simulink model "Button_bouncing"  (R2025b)
settings: Solver=VariableStepAuto  StartTime=0.0  StopTime=100  RelTol=1e-3
libraries: simulink x10, simulink_extras x2
settings Model: Creator=akame  LastModifiedBy=akame

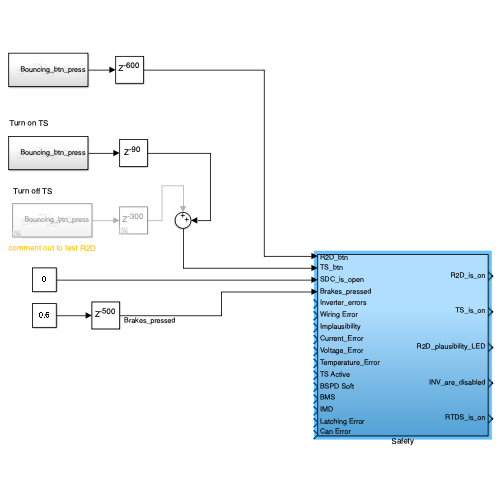
[thumbnail: Simulink's stored preview of the top-level diagram]
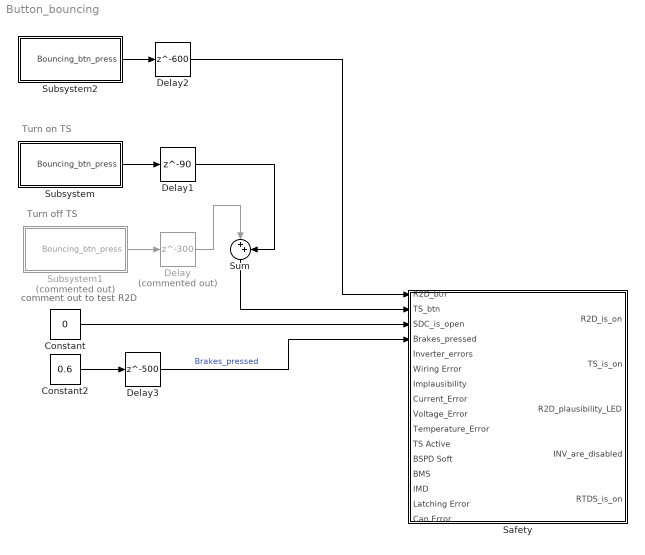
== system Button_bouncing ==
  note: Turn on TS
  note: Turn off TS
  note: comment out to test R2D
  Constant : Constant  Value=0
  Constant2 : Constant  Value=0.6
  Delay : Delay  Commented=on  DelayLength=300
  Delay1 : Delay  DelayLength=90
  Delay2 : Delay  DelayLength=600
  Delay3 : Delay  DelayLength=500
  Safety : Subsystem
  Subsystem : Subsystem
  Subsystem1 : Subsystem  Commented=on
  Subsystem2 : Subsystem
  Sum : Sum  Inputs=|++
  wires:
  Delay1/1 -> Sum/2
  Subsystem1/1(Bouncing_btn_press) -> Delay/1
  Subsystem/1(Bouncing_btn_press) -> Delay1/1
  Delay/1 -> Sum/1
  Sum/1 -> Safety/2(TS_btn)
  Constant/1 -> Safety/3(SDC_is_open)
  Subsystem2/1(Bouncing_btn_press) -> Delay2/1
  Delay2/1 -> Safety/1(R2D_btn)
  Constant2/1 -> Delay3/1
  Delay3/1 -> Safety/4(Brakes_pressed)  "Brakes_pressed"

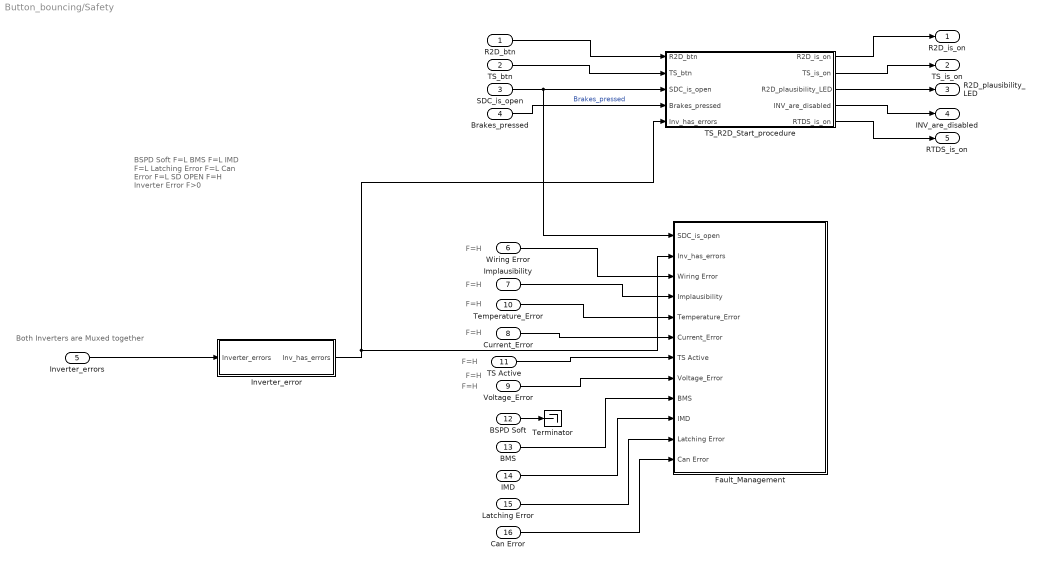
== system Button_bouncing/Safety ==
  note: Both Inverters are Muxed together
  note: F=H
  note: F=H
  note: F=H
  note: F=H
  note: F=H
  note: F=H
  note: F=H
  note: BSPD Soft		F=L
      | BMS			F=L
      | IMD				F=L
      | Latching Error	F=L
      | Can Error		F=L
      | SD OPEN		F=H
      | Inverter Error		F>0
  R2D_btn : Inport
  TS_btn : Inport  Port=2
  SDC_is_open : Inport  Port=3
  Brakes_pressed : Inport  Port=4
  Inverter_errors : Inport  Port=5
  Wiring Error : Inport  Port=6
  Implausibility : Inport  Port=7
  Current_Error : Inport  Port=8
  Voltage_Error : Inport  Port=9
  Temperature_Error : Inport  Port=10
  TS Active : Inport  Port=11
  BSPD Soft : Inport  Port=12
  BMS : Inport  Port=13
  IMD : Inport  Port=14
  Latching Error : Inport  Port=15
  Can Error : Inport  Port=16
  Fault_Management : Subsystem
  Inverter_error : Subsystem
  TS_R2D_Start_procedure : Subsystem
  Terminator : Terminator
  R2D_is_on : Outport
  TS_is_on : Outport  Port=2
  R2D_plausibility_LED : Outport  Port=3
  INV_are_disabled : Outport  Port=4
  RTDS_is_on : Outport  Port=5
  wires:
  TS_btn/1 -> TS_R2D_Start_procedure/2(TS_btn)
  SDC_is_open/1 -> Fault_Management/1(SDC_is_open), TS_R2D_Start_procedure/3(SDC_is_open)
  Brakes_pressed/1 -> TS_R2D_Start_procedure/4(Brakes_pressed)  "Brakes_pressed"
  R2D_btn/1 -> TS_R2D_Start_procedure/1(R2D_btn)
  Inverter_error/1(Inv_has_errors) -> Fault_Management/2(Inv_has_errors), TS_R2D_Start_procedure/5(Inv_has_errors)
  TS_R2D_Start_procedure/3(R2D_plausibility_LED) -> R2D_plausibility_LED/1
  TS_R2D_Start_procedure/1(R2D_is_on) -> R2D_is_on/1
  TS_R2D_Start_procedure/2(TS_is_on) -> TS_is_on/1
  TS_R2D_Start_procedure/4(INV_are_disabled) -> INV_are_disabled/1
  TS_R2D_Start_procedure/5(RTDS_is_on) -> RTDS_is_on/1
  TS Active/1 -> Fault_Management/7(TS Active)
  Wiring Error/1 -> Fault_Management/3(Wiring Error)
  Implausibility/1 -> Fault_Management/4(Implausibility)
  Current_Error/1 -> Fault_Management/6(Current_Error)
  Voltage_Error/1 -> Fault_Management/8(Voltage_Error)
  Temperature_Error/1 -> Fault_Management/5(Temperature_Error)
  Inverter_errors/1 -> Inverter_error/1(Inverter_errors)
  BMS/1 -> Fault_Management/9(BMS)
  IMD/1 -> Fault_Management/10(IMD)
  Latching Error/1 -> Fault_Management/11(Latching Error)
  Can Error/1 -> Fault_Management/12(Can Error)
  BSPD Soft/1 -> Terminator/1

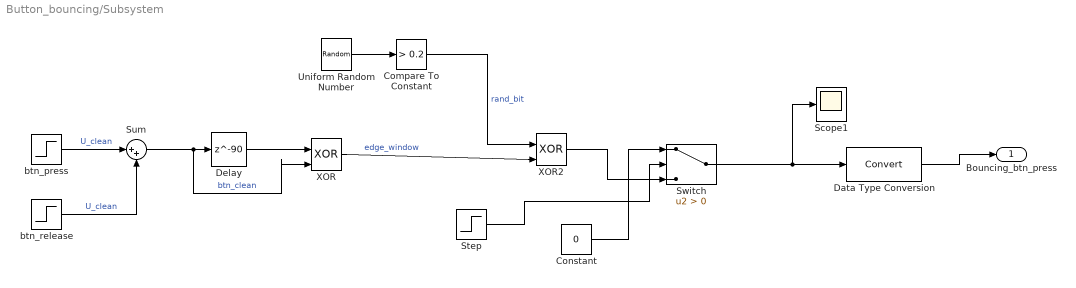
== system Button_bouncing/Subsystem ==
  Compare To Constant : simulink/Logic and Bit Operations/Compare To Constant  relop=>  const=0.2  OutDataTypeStr=boolean
  Constant : Constant  Value=0
  Data Type Conversion : DataTypeConversion  SaturateOnIntegerOverflow=off  RndMeth=Floor
  Delay : Delay  DelayLength=90
  Scope1 : Scope
      settings: ActiveDisplayYMinimum=-1  ActiveDisplayYMaximum=1  DataLoggingVariableName=ScopeData3
  Step : Step  Time=3  SampleTime=0
  Sum : Sum  Inputs=|++
  Switch : Switch  Criteria=u2 > Threshold  SaturateOnIntegerOverflow=off  InputSameDT=off
  Uniform Random Number : UniformRandomNumber  Minimum=0  SampleTime=0.1
  XOR : Logic  Operator=XOR  IconShape=distinctive  AllPortsSameDT=off  OutDataTypeStr=boolean
  XOR2 : Logic  Operator=XOR  IconShape=distinctive  AllPortsSameDT=off  OutDataTypeStr=boolean
  btn_press : Step  Time=0.05  SampleTime=0
  btn_release : Step  Time=0.15  After=-1  SampleTime=0
  Bouncing_btn_press : Outport
  wires:
  btn_press/1 -> Sum/1  "U_clean"
  btn_release/1 -> Sum/2  "U_clean"
  Sum/1 -> Delay/1, XOR/2  "btn_clean"
  Delay/1 -> XOR/1
  XOR/1 -> XOR2/2  "edge_window"
  Uniform Random Number/1 -> Compare To Constant/1
  Compare To Constant/1 -> XOR2/1  "rand_bit"
  Data Type Conversion/1 -> Bouncing_btn_press/1
  XOR2/1 -> Switch/3
  Switch/1 -> Data Type Conversion/1, Scope1/1
  Constant/1 -> Switch/1
  Step/1 -> Switch/2

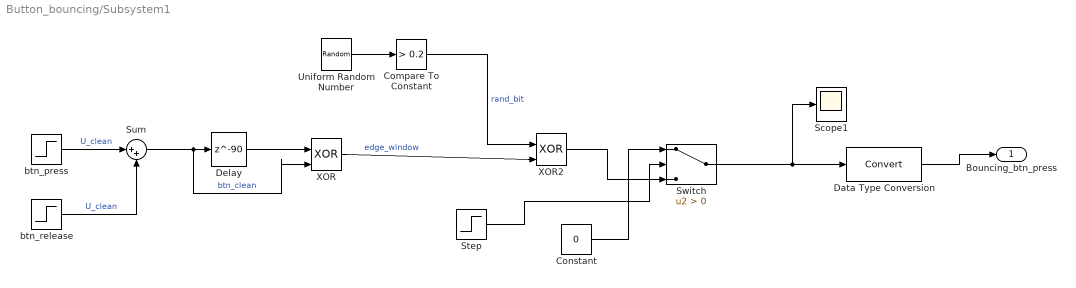
== system Button_bouncing/Subsystem1 ==
  Compare To Constant : simulink/Logic and Bit Operations/Compare To Constant  relop=>  const=0.2  OutDataTypeStr=boolean
  Constant : Constant  Value=0
  Data Type Conversion : DataTypeConversion  SaturateOnIntegerOverflow=off  RndMeth=Floor
  Delay : Delay  DelayLength=90
  Scope1 : Scope
      settings: ActiveDisplayYMinimum=-1  ActiveDisplayYMaximum=1  DataLoggingVariableName=ScopeData3
  Step : Step  Time=3  SampleTime=0
  Sum : Sum  Inputs=|++
  Switch : Switch  Criteria=u2 > Threshold  SaturateOnIntegerOverflow=off  InputSameDT=off
  Uniform Random Number : UniformRandomNumber  Minimum=0  SampleTime=0.1
  XOR : Logic  Operator=XOR  IconShape=distinctive  AllPortsSameDT=off  OutDataTypeStr=boolean
  XOR2 : Logic  Operator=XOR  IconShape=distinctive  AllPortsSameDT=off  OutDataTypeStr=boolean
  btn_press : Step  Time=0.05  SampleTime=0
  btn_release : Step  Time=0.15  After=-1  SampleTime=0
  Bouncing_btn_press : Outport
  wires:
  btn_press/1 -> Sum/1  "U_clean"
  btn_release/1 -> Sum/2  "U_clean"
  Sum/1 -> Delay/1, XOR/2  "btn_clean"
  Delay/1 -> XOR/1
  XOR/1 -> XOR2/2  "edge_window"
  Uniform Random Number/1 -> Compare To Constant/1
  Compare To Constant/1 -> XOR2/1  "rand_bit"
  Data Type Conversion/1 -> Bouncing_btn_press/1
  XOR2/1 -> Switch/3
  Switch/1 -> Data Type Conversion/1, Scope1/1
  Constant/1 -> Switch/1
  Step/1 -> Switch/2

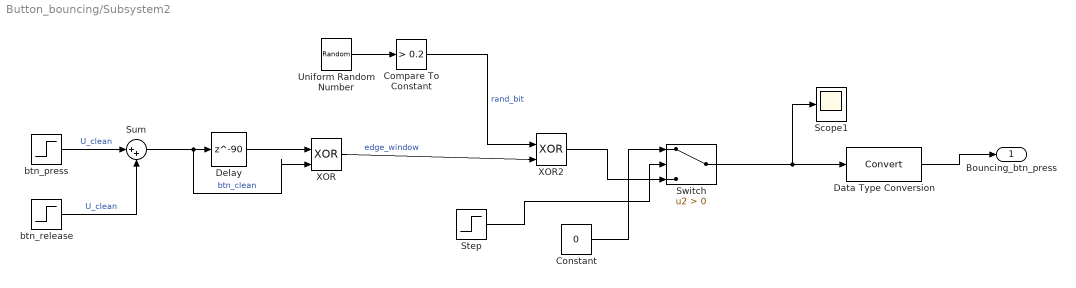
== system Button_bouncing/Subsystem2 ==
  Compare To Constant : simulink/Logic and Bit Operations/Compare To Constant  relop=>  const=0.2  OutDataTypeStr=boolean
  Constant : Constant  Value=0
  Data Type Conversion : DataTypeConversion  SaturateOnIntegerOverflow=off  RndMeth=Floor
  Delay : Delay  DelayLength=90
  Scope1 : Scope
      settings: ActiveDisplayYMinimum=-1  ActiveDisplayYMaximum=1  DataLoggingVariableName=ScopeData3
  Step : Step  Time=3  SampleTime=0
  Sum : Sum  Inputs=|++
  Switch : Switch  Criteria=u2 > Threshold  SaturateOnIntegerOverflow=off  InputSameDT=off
  Uniform Random Number : UniformRandomNumber  Minimum=0  SampleTime=0.1
  XOR : Logic  Operator=XOR  IconShape=distinctive  AllPortsSameDT=off  OutDataTypeStr=boolean
  XOR2 : Logic  Operator=XOR  IconShape=distinctive  AllPortsSameDT=off  OutDataTypeStr=boolean
  btn_press : Step  Time=0.05  SampleTime=0
  btn_release : Step  Time=0.15  After=-1  SampleTime=0
  Bouncing_btn_press : Outport
  wires:
  btn_press/1 -> Sum/1  "U_clean"
  btn_release/1 -> Sum/2  "U_clean"
  Sum/1 -> Delay/1, XOR/2  "btn_clean"
  Delay/1 -> XOR/1
  XOR/1 -> XOR2/2  "edge_window"
  Uniform Random Number/1 -> Compare To Constant/1
  Compare To Constant/1 -> XOR2/1  "rand_bit"
  Data Type Conversion/1 -> Bouncing_btn_press/1
  XOR2/1 -> Switch/3
  Switch/1 -> Data Type Conversion/1, Scope1/1
  Constant/1 -> Switch/1
  Step/1 -> Switch/2

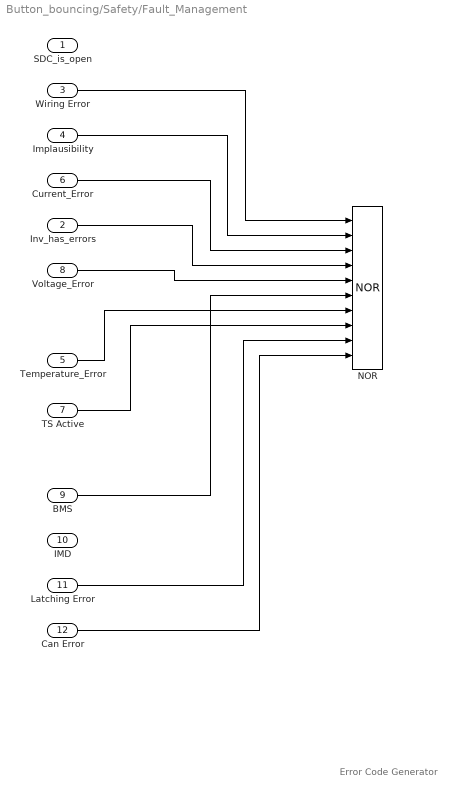
== system Button_bouncing/Safety/Fault_Management ==
  note: Error Code Generator
  SDC_is_open : Inport
  Inv_has_errors : Inport  Port=2
  Wiring Error : Inport  Port=3
  Implausibility : Inport  Port=4
  Temperature_Error : Inport  Port=5
  Current_Error : Inport  Port=6
  TS Active : Inport  Port=7
  Voltage_Error : Inport  Port=8
  BMS : Inport  Port=9
  IMD : Inport  Port=10
  Latching Error : Inport  Port=11
  Can Error : Inport  Port=12
  NOR : Logic  Operator=NOR  Inputs=10  AllPortsSameDT=off  OutDataTypeStr=boolean
  wires:
  Wiring Error/1 -> NOR/1
  Implausibility/1 -> NOR/2
  Current_Error/1 -> NOR/3
  Voltage_Error/1 -> NOR/5
  Temperature_Error/1 -> NOR/7
  TS Active/1 -> NOR/8
  Inv_has_errors/1 -> NOR/4
  Can Error/1 -> NOR/10
  Latching Error/1 -> NOR/9
  BMS/1 -> NOR/6

== system Button_bouncing/Safety/Inverter_error ==
  note: Check if Error codes are more than 0
  Inverter_errors : Inport
  Compare To Constant : simulink/Logic and Bit Operations/Compare To Constant  relop=>  const=0  OutDataTypeStr=boolean
  Compare To Constant1 : simulink/Logic and Bit Operations/Compare To Constant  relop=>  const=0  OutDataTypeStr=boolean
  Demux : Demux  Outputs=2
  Inv_has_errors : Outport
  wires:
  Inverter_errors/1 -> Demux/1
  Demux/1 -> Compare To Constant/1
  Demux/2 -> Compare To Constant1/1

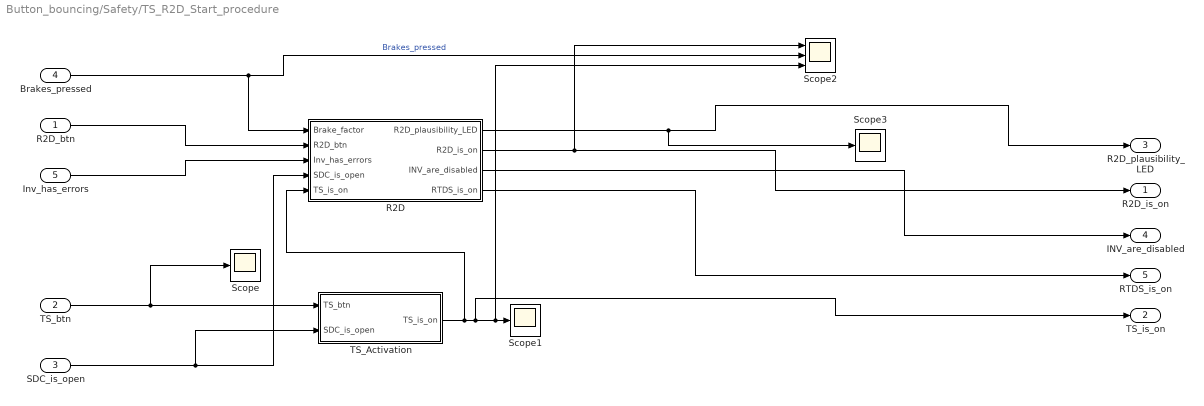
== system Button_bouncing/Safety/TS_R2D_Start_procedure ==
  R2D_btn : Inport
  TS_btn : Inport  Port=2
  SDC_is_open : Inport  Port=3
  Brakes_pressed : Inport  Port=4
  Inv_has_errors : Inport  Port=5
  R2D : Subsystem
  Scope : Scope
      settings: ActiveDisplayYMinimum=-0.14271551234259128  ActiveDisplayYMaximum=1.0309109576539348  DataLoggingVariableName=ScopeData9
  Scope1 : Scope
      settings: ActiveDisplayYMinimum=-1  ActiveDisplayYMaximum=1  DataLoggingVariableName=ScopeData10
  Scope2 : Scope  NumInputPorts=3
      settings: ActiveDisplayYMinimum=-0.12499999999999997  ActiveDisplayYMaximum=1.125  DataLoggingVariableName=ScopeData11
  Scope3 : Scope
      settings: ActiveDisplayYMinimum=-1  ActiveDisplayYMaximum=1  DataLoggingVariableName=ScopeData12
  TS_Activation : Subsystem
  R2D_is_on : Outport
  TS_is_on : Outport  Port=2
  R2D_plausibility_LED : Outport  Port=3
  INV_are_disabled : Outport  Port=4
  RTDS_is_on : Outport  Port=5
  wires:
  Brakes_pressed/1 -> Scope2/2, R2D/1(Brake_factor)  "Brakes_pressed"
  R2D/2(R2D_is_on) -> R2D_is_on/1, Scope2/1
  Inv_has_errors/1 -> R2D/3(Inv_has_errors)
  R2D_btn/1 -> R2D/2(R2D_btn)
  R2D/4(RTDS_is_on) -> RTDS_is_on/1
  TS_btn/1 -> Scope/1, TS_Activation/1(TS_btn)
  R2D/3(INV_are_disabled) -> INV_are_disabled/1
  R2D/1(R2D_plausibility_LED) -> R2D_plausibility_LED/1, Scope3/1
  TS_Activation/1(TS_is_on) -> Scope2/3, Scope1/1, TS_is_on/1, R2D/5(TS_is_on)
  SDC_is_open/1 -> R2D/4(SDC_is_open), TS_Activation/2(SDC_is_open)

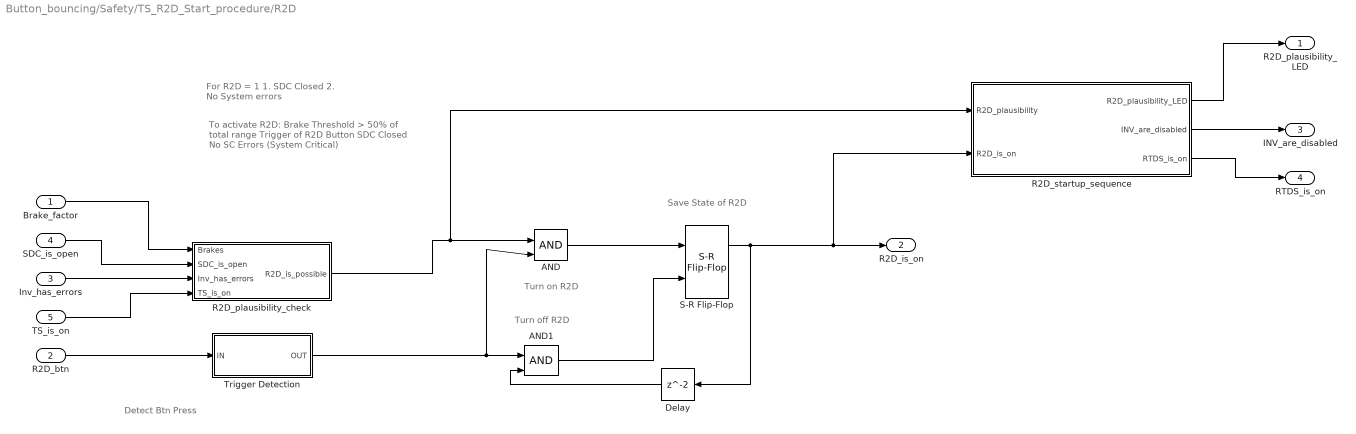
== system Button_bouncing/Safety/TS_R2D_Start_procedure/R2D ==
  note: Turn on R2D
  note: Turn off R2D
  note: Detect Btn Press
  note: Save State of R2D
  note: To activate R2D:
      | Brake Threshold > 50% of total range
      | Trigger of R2D Button
      | SDC Closed
      | No SC Errors (System Critical)
  note: For R2D = 1
      |  1. SDC Closed
      |  2. No System errors
  Brake_factor : Inport
  R2D_btn : Inport  Port=2
  Inv_has_errors : Inport  Port=3
  SDC_is_open : Inport  Port=4
  TS_is_on : Inport  Port=5
  AND : Logic  IconShape=distinctive  AllPortsSameDT=off  OutDataTypeStr=boolean
  AND1 : Logic  IconShape=distinctive  AllPortsSameDT=off  OutDataTypeStr=boolean
  Delay : Delay
  R2D_plausibility_check : Subsystem
  R2D_startup_sequence : Subsystem
  S-R Flip-Flop : simulink_extras/Flip Flops/S-R Flip-Flop  initial_condition=0
  Trigger Detection : Subsystem
  R2D_plausibility_LED : Outport
  R2D_is_on : Outport  Port=2
  INV_are_disabled : Outport  Port=3
  RTDS_is_on : Outport  Port=4
  wires:
  R2D_btn/1 -> Trigger Detection/1(IN)
  Trigger Detection/1(OUT) -> AND1/1, AND/2
  AND/1 -> S-R Flip-Flop/1
  AND1/1 -> S-R Flip-Flop/2
  Brake_factor/1 -> R2D_plausibility_check/1(Brakes)
  SDC_is_open/1 -> R2D_plausibility_check/2(SDC_is_open)
  Inv_has_errors/1 -> R2D_plausibility_check/3(Inv_has_errors)
  R2D_plausibility_check/1(R2D_is_possible) -> R2D_startup_sequence/1(R2D_plausibility), AND/1
  TS_is_on/1 -> R2D_plausibility_check/4(TS_is_on)
  Delay/1 -> AND1/2
  S-R Flip-Flop/1 -> R2D_startup_sequence/2(R2D_is_on), R2D_is_on/1, Delay/1
  R2D_startup_sequence/1(R2D_plausibility_LED) -> R2D_plausibility_LED/1
  R2D_startup_sequence/2(INV_are_disabled) -> INV_are_disabled/1
  R2D_startup_sequence/3(RTDS_is_on) -> RTDS_is_on/1

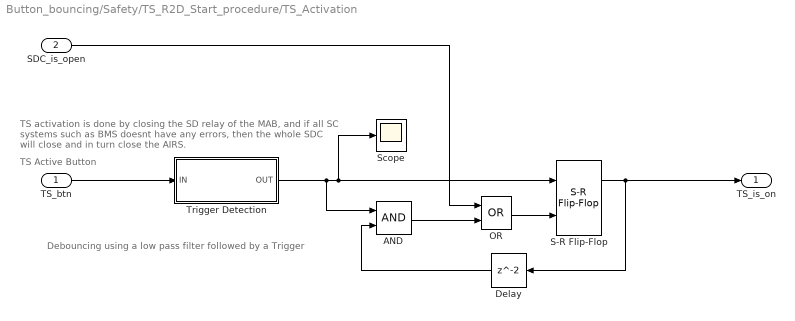
== system Button_bouncing/Safety/TS_R2D_Start_procedure/TS_Activation ==
  note: TS activation is done by closing the SD relay of the MAB,
      | and if all SC systems such as BMS doesnt have any errors, then
      | the whole SDC will close and in turn close the AIRS.
  note: TS Active Button
  note: Debouncing using a low pass filter followed by a Trigger
  TS_btn : Inport
  SDC_is_open : Inport  Port=2
  AND : Logic  AllPortsSameDT=off  OutDataTypeStr=boolean
  Delay : Delay
  OR : Logic  Operator=OR  AllPortsSameDT=off  OutDataTypeStr=boolean
  S-R Flip-Flop : simulink_extras/Flip Flops/S-R Flip-Flop  initial_condition=0
  Scope : Scope
      settings: ActiveDisplayYMinimum=-1  ActiveDisplayYMaximum=1
  Trigger Detection : Subsystem
  TS_is_on : Outport
  wires:
  S-R Flip-Flop/1 -> Delay/1, TS_is_on/1
  Trigger Detection/1(OUT) -> S-R Flip-Flop/1, Scope/1, AND/1
  OR/1 -> S-R Flip-Flop/2
  AND/1 -> OR/2
  TS_btn/1 -> Trigger Detection/1(IN)
  SDC_is_open/1 -> OR/1
  Delay/1 -> AND/2

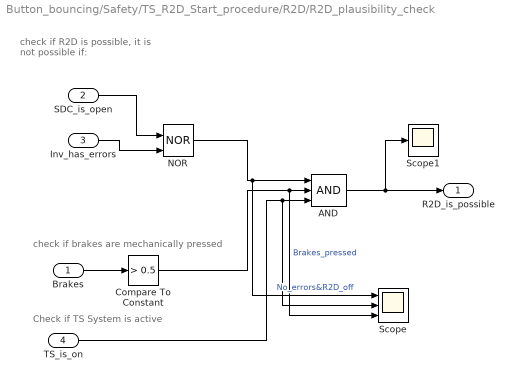
== system Button_bouncing/Safety/TS_R2D_Start_procedure/R2D/R2D_plausibility_check ==
  note: Check if TS System is active
  note: check if brakes are mechanically pressed
  note: check if R2D is possible,
      | it is not possible if:
  Brakes : Inport
  SDC_is_open : Inport  Port=2
  Inv_has_errors : Inport  Port=3
  TS_is_on : Inport  Port=4
  AND : Logic  Inputs=3  IconShape=distinctive  AllPortsSameDT=off  OutDataTypeStr=boolean
  Compare To Constant : simulink/Logic and Bit Operations/Compare To Constant  relop=>  const=0.5  OutDataTypeStr=boolean
  NOR : Logic  Operator=NOR  IconShape=distinctive  AllPortsSameDT=off  OutDataTypeStr=boolean
  Scope : Scope  NumInputPorts=3
      settings: ActiveDisplayYMinimum=-0.12499999999999997  ActiveDisplayYMaximum=1.125  DataLoggingVariableName=ScopeData5
  Scope1 : Scope
      settings: ActiveDisplayYMinimum=-1  ActiveDisplayYMaximum=1  DataLoggingVariableName=ScopeData6
  R2D_is_possible : Outport
  wires:
  Brakes/1 -> Compare To Constant/1
  Compare To Constant/1 -> Scope/3, AND/2  "Brakes_pressed"
  Inv_has_errors/1 -> NOR/2
  SDC_is_open/1 -> NOR/1
  NOR/1 -> Scope/1, AND/1  "No_errors&R2D_off"
  AND/1 -> Scope1/1, R2D_is_possible/1
  TS_is_on/1 -> Scope/2, AND/3

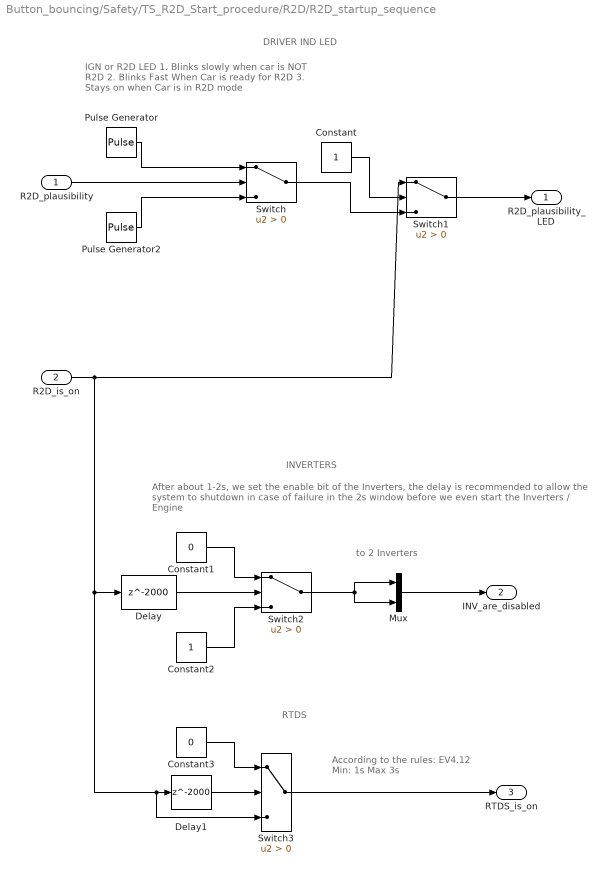
== system Button_bouncing/Safety/TS_R2D_Start_procedure/R2D/R2D_startup_sequence ==
  note: INVERTERS
  note: According to the rules: EV4.12
      | Min: 1s
      | Max 3s
  note: to 2 Inverters
  note: After about 1-2s, we set the enable bit of the Inverters,
      |
      | the delay is recommended to allow the system to shutdown in case of failure in the 2s window before we even start the Inverters / Engine
  note: IGN or R2D LED
      | 	1. Blinks slowly when car is NOT R2D
      | 	2. Blinks Fast When Car is ready for R2D
      | 	3. Stays on when Car is in R2D mode
  note: RTDS
  note: DRIVER IND LED
  R2D_plausibility : Inport
  R2D_is_on : Inport  Port=2
  Constant : Constant
  Constant1 : Constant  Value=0
  Constant2 : Constant
  Constant3 : Constant  Value=0
  Delay : Delay  DelayLength=2000
  Delay1 : Delay  DelayLength=2000
  Mux : Mux  Inputs=2
  Pulse Generator : DiscretePulseGenerator  PulseType=Time based  Period=0.5  PulseWidth=50
  Pulse Generator2 : DiscretePulseGenerator  PulseType=Time based  PulseWidth=12.5
  Switch{,1..3} (4 alike) : Switch  Criteria=u2 > Threshold  SaturateOnIntegerOverflow=off  InputSameDT=off
  R2D_plausibility_LED : Outport
  INV_are_disabled : Outport  Port=2
  RTDS_is_on : Outport  Port=3
  wires:
  Switch/1 -> Switch1/3
  Pulse Generator/1 -> Switch/1
  Pulse Generator2/1 -> Switch/3
  R2D_plausibility/1 -> Switch/2
  R2D_is_on/1 -> Switch3/3, Delay1/1, Delay/1, Switch1/1
  Constant/1 -> Switch1/2
  Switch1/1 -> R2D_plausibility_LED/1
  Delay/1 -> Switch2/2
  Constant1/1 -> Switch2/1
  Constant2/1 -> Switch2/3
  Switch2/1 -> Mux/1, Mux/2
  Mux/1 -> INV_are_disabled/1
  Delay1/1 -> Switch3/2
  Constant3/1 -> Switch3/1
  Switch3/1 -> RTDS_is_on/1

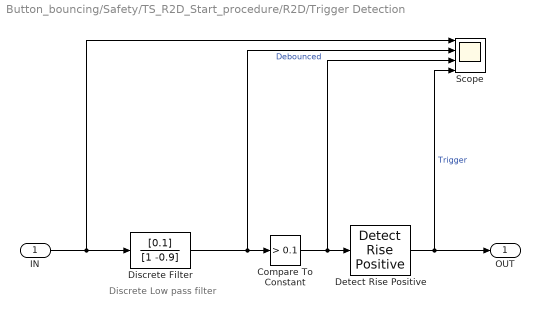
== system Button_bouncing/Safety/TS_R2D_Start_procedure/R2D/Trigger Detection ==
  note: Discrete Low pass filter
  IN : Inport
  Compare To Constant : simulink/Logic and Bit Operations/Compare To Constant  relop=>  const=0.1  OutDataTypeStr=boolean
  Detect Rise Positive : simulink/Logic and Bit Operations/Detect Rise Positive  vinit=0  OutDataTypeStr=boolean
  Discrete Filter : DiscreteFilter  Numerator=[0.1]  Denominator=[1 -0.9]
  Scope : Scope  NumInputPorts=4
      settings: ActiveDisplayYMinimum=-0.020414905821153462  ActiveDisplayYMaximum=1.0278629493510638  DataLoggingVariableName=ScopeData2
  OUT : Outport
  wires:
  IN/1 -> Discrete Filter/1, Scope/1
  Compare To Constant/1 -> Scope/3, Detect Rise Positive/1
  Discrete Filter/1 -> Scope/2, Compare To Constant/1  "Debounced"
  Detect Rise Positive/1 -> Scope/4, OUT/1  "Trigger"

== system Button_bouncing/Safety/TS_R2D_Start_procedure/TS_Activation/Trigger Detection ==
  note: Discrete Low pass filter
  IN : Inport
  Compare To Constant : simulink/Logic and Bit Operations/Compare To Constant  relop=>  const=0.1  OutDataTypeStr=boolean
  Detect Rise Positive : simulink/Logic and Bit Operations/Detect Rise Positive  vinit=0  OutDataTypeStr=boolean
  Discrete Filter : DiscreteFilter  Numerator=[0.1]  Denominator=[1 -0.9]
  Scope : Scope  NumInputPorts=4
      settings: ActiveDisplayYMinimum=0.0009331921028933321  ActiveDisplayYMaximum=0.797393918699171  DataLoggingVariableName=ScopeData2
  OUT : Outport
  wires:
  IN/1 -> Discrete Filter/1, Scope/1
  Compare To Constant/1 -> Scope/3, Detect Rise Positive/1
  Discrete Filter/1 -> Scope/2, Compare To Constant/1  "Debounced"
  Detect Rise Positive/1 -> Scope/4, OUT/1  "Trigger"
